simulink model "Terceiro_Trabalho"  (R2015a)
settings: Solver=ode45  StartTime=0.0  StopTime=10  RelTol=1e-3
libraries: simulink x1
settings Model: Creator=kreislerb  LastModifiedBy=kreislerb

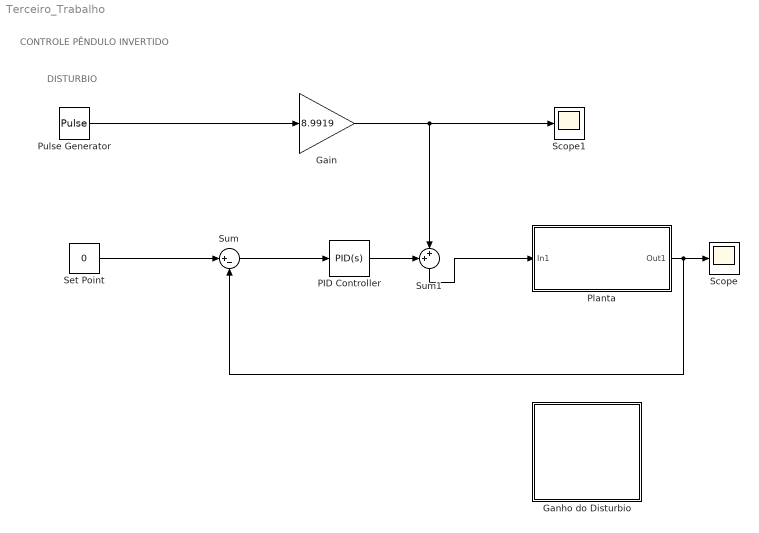
== system Terceiro_Trabalho ==
  note: CONTROLE PÊNDULO INVERTIDO
  note: DISTURBIO
  "Gain " : Gain  Gain=8.9919  OutMin=[-30]  OutMax=[30]
  Ganho do Disturbio : Subsystem  DialogController=hmiCreateDDGDialog  IsWebBlock=on  mask(MathWorksWebBlock){webBlockId=00d170c9-ed68-4c8d-904c-7865c277f6cd, webBlockType=continuousknob, ShowInLibBrowser=on, ShowInitialText=on, HMISrcModelName=Terceiro_Trabalho}
      mask prompts: webBlockId "WebBlock Id"; webBlockType "WebBlock Type"; HMISrcModelName "Source Model"
      mask Help: helpview([docroot '/mapfiles/simulink.map'], 'hmi_knob')
      mask Display:
      | if strcmp(get_param(bdroot(gcb),'BlockDiagramType'), 'library')
      |     image([(matlabroot) '/toolbox/simulink/hmi/icons/ContinuousKnob.png']);
      | end
  PID Controller : simulink/Continuous/PID Controller  Controller=PID  TimeDomain=Continuous-time  SampleTime=-1  IntegratorMethod=Forward Euler  FilterMethod=Forward Euler  Form=Parallel  UseFilter=on  ControllerParametersSource=internal  P=1671.20520393919  I=2463.33206421087  D=278.40683130766  N=171.720828335783  InitialConditionSource=internal  InitialConditionForIntegrator=0  InitialConditionForFilter=0  ExternalReset=none  LimitOutput=off  UpperSaturationLimit=inf  LowerSaturationLimit=-inf  LinearizeAsGain=on  AntiWindupMode=none  Kb=1  TrackingMode=off  Kt=1  PParamMin=[]  PParamMax=[]  IParamMin=[]  IParamMax=[]  DParamMin=[]  DParamMax=[]  NParamMin=[]  NParamMax=[]  KbParamMin=[]  KbParamMax=[]  KtParamMin=[]  KtParamMax=[]  POutMin=[]  POutMax=[]  IOutMin=[]  IOutMax=[]  DOutMin=[]  DOutMax=[]  NOutMin=[]  NOutMax=[]  KbOutMin=[]  KbOutMax=[]  KtOutMin=[]  KtOutMax=[]  IntegratorOutMin=[]  IntegratorOutMax=[]  FilterOutMin=[]  FilterOutMax=[]  SumOutMin=[]  SumOutMax=[]  SumI1OutMin=[]  SumI1OutMax=[]  SumI2OutMin=[]  SumI2OutMax=[]  SumI3OutMin=[]  SumI3OutMax=[]  SumDOutMin=[]  SumDOutMax=[]  SaturationOutMin=[]  SaturationOutMax=[]  IntegratorContinuousStateAttributes=''  IntegratorStateMustResolveToSignalObject=off  IntegratorRTWStateStorageClass=Auto  FilterContinuousStateAttributes=''  FilterStateMustResolveToSignalObject=off  FilterRTWStateStorageClass=Auto  DifferentiatorICPrevScaledInput=0  DifferentiatorOutMin=[]  DifferentiatorOutMax=[]
  Planta : Subsystem  mask{Mc=3, l=3, m=5, g=9.81}
      mask prompts: Mc "Massa do Carro(Mc)"; l "Distancia do CM (l)"; m "Massa do Pendulo (m)"; g "Aceleração gravitacional (g)"
      mask help: Função de transferência de um pêndulo invertido com centro de massa na extremidade superior
  Pulse Generator : DiscretePulseGenerator  PulseType=Time based  Period=3  PulseWidth=0.01  SampleTime=10
  Scope : Scope
      settings: TimeRange=10  YMin=-2e-07  YMax=9e-07
  Scope1 : Scope
      settings: TimeRange=10  YMin=4.3805  YMax=4.3805
  Set Point : Constant  Value=0
  Sum : Sum  Inputs=|+-
  Sum1 : Sum  Inputs=++|
  wires:
  Sum/1 -> PID Controller/1
  Set Point/1 -> Sum/1
  "Gain "/1 -> Sum1/2, Scope1/1
  Pulse Generator/1 -> "Gain "/1
  PID Controller/1 -> Sum1/1
  Sum1/1 -> Planta/1(In1)
  Planta/1(Out1) -> Scope/1, Sum/2

== system Terceiro_Trabalho/Ganho do Disturbio ==

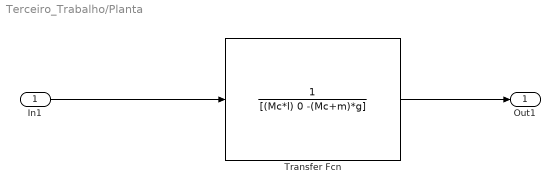
== system Terceiro_Trabalho/Planta ==
  In1 : Inport
  Transfer Fcn : TransferFcn  Denominator=[(Mc*l) 0 -(Mc+m)*g]
  Out1 : Outport
  wires:
  In1/1 -> Transfer Fcn/1
  Transfer Fcn/1 -> Out1/1
